simulink model "NEWCKT"  (R2021b)
settings: Solver=VariableStepAuto  StartTime=0.0  StopTime=10.0  RelTol=1e-3
undefined symbols (not defined in the file): Ion, Lithium
libraries: spsIdealSwitchLib x3, spsBatteryLib x2, spsSeriesRLCBranchLib x1, spspowerguiLib x1
settings Model: Creator=Admin  LastModifiedBy=Admin
settings ConfigComp: CovScope=ReferencedModels

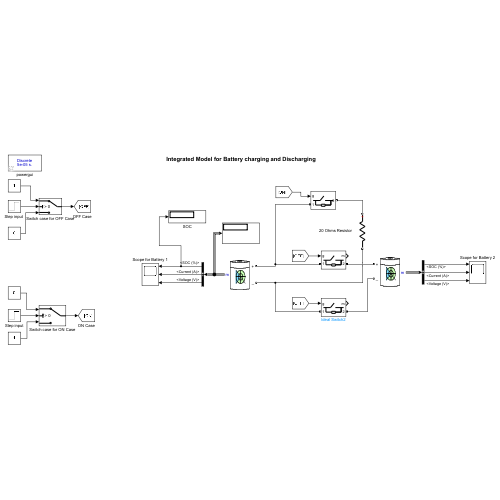
[thumbnail: Simulink's stored preview of the top-level diagram]
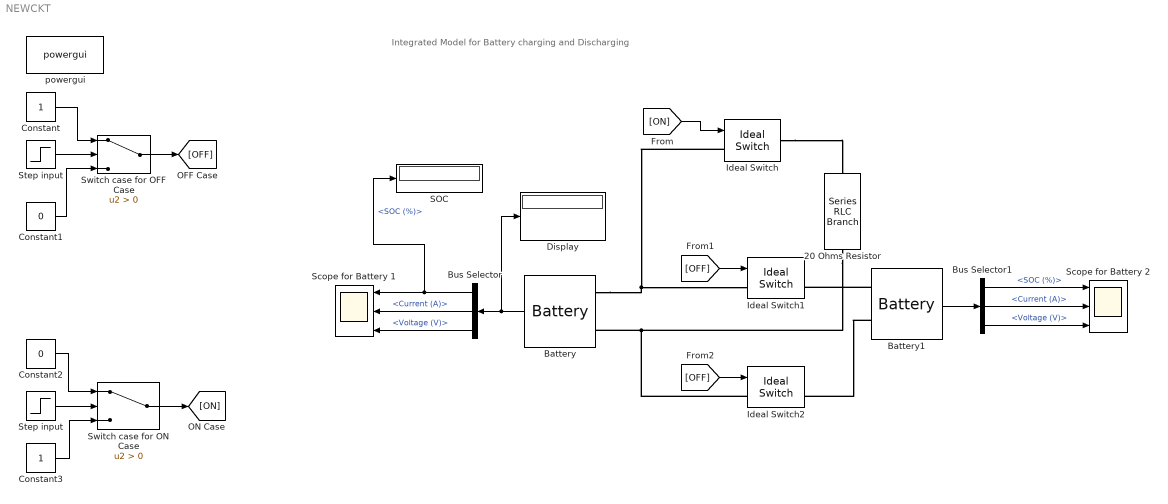
== system NEWCKT ==
  note: Integrated Model for Battery charging and Discharging
  20 Ohms Resistor : spsSeriesRLCBranchLib/Series RLC Branch  LConnTagsString=__new0  RConnTagsString=__new0  BranchType=R  Resistance=20  Inductance=1e-3  SetiL0=off  InitialCurrent=0  Capacitance=1e-6  Setx0=off  InitialVoltage=0  Measurements=None
  Battery : spsBatteryLib/Battery  BatType=Lithium-Ion  ShowTempParam=off  ThermalPreset=no  ShowAgeParam=off  NomV=7.2  NomQ=5.4  SOC=80  Batt_Tr=30  PresetModel=on  MaxQ=5.4  MinV=5.4  FullV=8.3807  Dis_rate=2.3478  R=0.013333  Normal_OP=4.8835  expZone="[7.7788      0.2653]"  current=[6.5 13 32.5]  Units=Time  Tci=20  NomT=20  T2=-30  MaxQ2=4.8  FullV2=7.1  Normal_OP2=5.655  expZone2="[6.58           1]"  Rca=0.6  ti=2000  Dp=0  Neq0=0  Tsim=1e6  Ta1=25  Qeol=5.4*0.9  Reol=0.013333*1.2  Char_age=[2.3478, 3]  Dis_age=[2.3478, 10]  N1=1500  N2=10500  N3=1000  N4=1400  Ta2=45  N5=950
  Battery1 : spsBatteryLib/Battery  BatType=Lithium-Ion  ShowTempParam=off  ThermalPreset=no  ShowAgeParam=off  NomV=7.2  NomQ=5.4  SOC=100  Batt_Tr=30  PresetModel=on  MaxQ=5.4  MinV=5.4  FullV=8.3807  Dis_rate=2.3478  R=0.013333  Normal_OP=4.8835  expZone="[7.7788      0.2653]"  current=[6.5 13 32.5]  Units=Time  Tci=20  NomT=20  T2=-30  MaxQ2=4.8  FullV2=7.1  Normal_OP2=5.655  expZone2="[6.58           1]"  Rca=0.6  ti=2000  Dp=0  Neq0=0  Tsim=1e6  Ta1=25  Qeol=5.4*0.9  Reol=0.013333*1.2  Char_age=[2.3478, 3]  Dis_age=[2.3478, 10]  N1=1500  N2=10500  N3=1000  N4=1400  Ta2=45  N5=950
  Bus Selector : BusSelector  OutputSignals=SOC (%),Current (A),Voltage (V)
  Bus Selector1 : BusSelector  OutputSignals=SOC (%),Current (A),Voltage (V)
  Constant : Constant
  Constant1 : Constant  Value=0
  Constant2 : Constant  Value=0
  Constant3 : Constant
  Display : Display
  Ideal Switch : spsIdealSwitchLib/Ideal Switch  Ron=0.001  Lon=0  IC=0  Rs=1e5  Cs=inf  Measurements=off
  Ideal Switch1 : spsIdealSwitchLib/Ideal Switch  Ron=0.001  Lon=0  IC=0  Rs=1e5  Cs=inf  Measurements=on
  Ideal Switch2 : spsIdealSwitchLib/Ideal Switch  Ron=0.001  Lon=0  IC=0  Rs=1e5  Cs=inf  Measurements=on
  SOC : Display
  Scope for Battery 1 : Scope  NumInputPorts=3
  Scope for Battery 2 : Scope  NumInputPorts=3
  Step input : Step  Time=4  SampleTime=0
  "Step input " : Step  Time=4  SampleTime=0
  Switch case for OFF Case : Switch  Criteria=u2 > Threshold
  Switch case for ON Case : Switch  Criteria=u2 > Threshold
  powergui : spspowerguiLib/powergui  Priority=1  SimulationMode=Discrete  SampleTime=50e-6  frequency=60  Iterations=50  frequencyindice=0  Pbase=100e6  ErrMax=1e-4  UnitsV=kV  UnitsW=MW  buscounter=0  FunctionMessages=off  echomessages=off  EnableUseOfTLC=off  CurrentSourceSwitches=off  DisableSnubberDevices=off  DisableRonSwitches=off  DisableVfSwitches=off  DisplayEquations=off  AutomaticDiscreteSolvers=off  SolverType=Tustin/Backward Euler (TBE)  Interpol=off  ExternalGateDelay=off  methode=off  Ts=100  x0status=blocks  SPID=on  SwTol=0  HookPort=off  NonlinearTolerance=1e-4  nMaxIteration=100  ContinueOnMaxIteration=off  RestoreLinks=warning  ResistiveCurrentMeasurement=off  Frange=[0:2:500]  Ylog=off  Xlog=on  ShowGrid=off  save=off  variable=ZData  structure=0  ZoomFFT=off  StartTime=0.0  cycles=1  DisplayStyle=1  fundamental=60  FreqAxis=off  MaxFrequency=1000  frequencyindicesteady=1  RmsSteady=1  display=off
  wires:
  Battery/1 -> Display/1, Bus Selector/1
  Bus Selector/2 -> Scope for Battery 1/2  "<Current (A)>"
  Bus Selector/1 -> SOC/1, Scope for Battery 1/1  "<SOC (%)>"
  "Step input "/1 -> Switch case for OFF Case/2
  Constant/1 -> Switch case for OFF Case/1
  Constant1/1 -> Switch case for OFF Case/3
  Constant2/1 -> Switch case for ON Case/1
  Constant3/1 -> Switch case for ON Case/3
  Step input/1 -> Switch case for ON Case/2
  Bus Selector/3 -> Scope for Battery 1/3  "<Voltage (V)>"
  Switch case for OFF Case/1 -> [OFF]
  Switch case for ON Case/1 -> [ON]
  [ON] -> Ideal Switch/1
  [OFF] -> Ideal Switch2/1
  [OFF] -> Ideal Switch1/1
  Battery1/1 -> Bus Selector1/1
  Bus Selector1/1 -> Scope for Battery 2/1  "<SOC (%)>"
  Bus Selector1/2 -> Scope for Battery 2/2  "<Current (A)>"
  Bus Selector1/3 -> Scope for Battery 2/3  "<Voltage (V)>"
  connections:
  Ideal Switch/RConn1 -- 20 Ohms Resistor/LConn1
  Battery1/LConn1 -- Ideal Switch1/RConn1
  Battery1/LConn2 -- Ideal Switch2/RConn1
  Ideal Switch2/LConn1 -- 20 Ohms Resistor/RConn1 -- Battery/LConn2
  Battery/LConn1 -- Ideal Switch/LConn1 -- Ideal Switch1/LConn1
